simulink subsystem "Subsystem_DCmotor"  (R2021a)
settings: Solver=VariableStepAuto  StartTime=0.0  StopTime=10.0  RelTol=1e-3
values from neighbouring files (symbols this model uses):
  B1 = I1^2*(B)    (= 0.000841892548715)    [parameters.m]
  I1 = 36    [parameters.m]
  J1 = I1^2*(J+J_gear)+J_arm    (= 0.002471936)    [parameters.m]
  Kb = 9.73*10^-3    (= 0.00973)    [parameters.m]
  Km = 9.73*10^-3    (= 0.00973)    [parameters.m]
  L = 0.035*10^-3    (= 3.5e-05)    [parameters.m]
  R = 0.335    [parameters.m]
settings Model: Creator=czq80  LastModifiedBy=czq80
settings SolverCC: AlgebraicLoopSolver=TrustRegion
settings DebuggingCC: SFMachineParentedDataDiag=warning

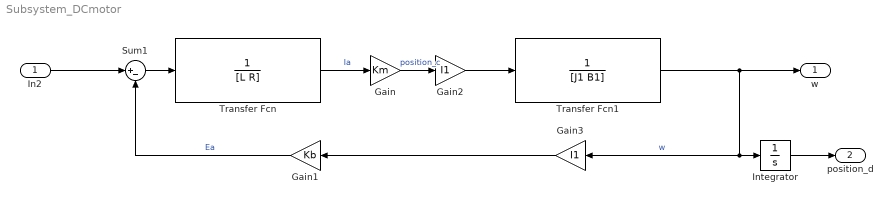
== system Subsystem_DCmotor ==
  In2 : Inport
  Gain : Gain  Gain=Km
  Gain1 : Gain  Gain=Kb
  Gain2 : Gain  Gain=I1
  Gain3 : Gain  Gain=I1
  Integrator : Integrator
  Sum1 : Sum  Inputs=|+-
  Transfer Fcn : TransferFcn  Denominator=[L R]
  Transfer Fcn1 : TransferFcn  Denominator=[J1 B1]
  w : Outport
  position_d : Outport  Port=2
  wires:
  Sum1/1 -> Transfer Fcn/1
  Transfer Fcn/1 -> Gain/1  "Ia"
  Gain1/1 -> Sum1/2  "Ea"
  Transfer Fcn1/1 -> w/1, Integrator/1, Gain3/1  "w"
  In2/1 -> Sum1/1
  Integrator/1 -> position_d/1
  Gain/1 -> Gain2/1  "position_c"
  Gain2/1 -> Transfer Fcn1/1
  Gain3/1 -> Gain1/1
